simulink model "bare_system"  (Simulink 9.3)
settings: Solver=VariableStepAuto  StartTime=0.0  StopTime=stopTime  RelTol=1e-3
model workspace (MAT data in the model file):
  avg_usersArg = Simulink.Parameter
  avg_usersArg.Value = 4
  avg_usersArg.DataType = 'auto'
  avg_usersArg.Dimensions = [1 1]
  lambda1Arg = Simulink.Parameter
  lambda1Arg.Value = 1
  lambda1Arg.DataType = 'auto'
  lambda1Arg.Dimensions = [1 1]
  lambda2Arg = Simulink.Parameter
  lambda2Arg.Value = 1
  lambda2Arg.DataType = 'auto'
  lambda2Arg.Dimensions = [1 1]
  lower_limitArg = Simulink.Parameter
  lower_limitArg.Value = 1
  lower_limitArg.DataType = 'auto'
  lower_limitArg.Dimensions = [1 1]
  random_seedArg = Simulink.Parameter
  random_seedArg.Value = 1
  random_seedArg.DataType = 'auto'
  random_seedArg.Dimensions = [1 1]
  risk_delayArg = Simulink.Parameter
  risk_delayArg.Value = 1
  risk_delayArg.DataType = 'auto'
  risk_delayArg.Dimensions = [1 1]
  risk_delay_lengthArg = Simulink.Parameter
  risk_delay_lengthArg.Value = 1
  risk_delay_lengthArg.DataType = 'auto'
  risk_delay_lengthArg.Dimensions = [1 1]
  upper_limitArg = Simulink.Parameter
  upper_limitArg.Value = 1
  upper_limitArg.DataType = 'auto'
  upper_limitArg.Dimensions = [1 1]
values from neighbouring files (symbols this model uses):
  delta = 1e-10    [initParamsDefault.m]
  interval = 1    [train_ddpg.m]    (also in train_dqn.m)
  is_done_limit = 1200    [initParamsDefault.m]
  l1_cf = 2.4    [initParamsDefault.m]
  l1_ig = 1.5    [initParamsDefault.m]
  n = numel(vectors)    [initParamsDefault.m]
  omega = 0.1    [initParamsDefault.m]
  Pexec = 5    [initParamsDefault.m]
  Pidle = 0.1    [initParamsDefault.m]
  Ptx = 1    [initParamsDefault.m]
  Rate = [ ... (first row only)    [WIFI_speeds.m]
  sample_time = 0.1    [train_ddpg.m]    (also in train_dqn.m)
  stopTime = 40    [train_ddpg.m]    (also in train_dqn.m)
  tau_threshold = 5    [initParamsDefault.m]
  w_completion = 0.01    [initParamsDefault.m]
  w_drop = 1    [initParamsDefault.m]
  w_e = 0.5    [initParamsDefault.m]
  w_r = 1    [initParamsDefault.m]
  w_t = 0.1    [initParamsDefault.m]
undefined symbols (not defined in the file or in its folder): G11, G21, m
libraries: dspswit3 x2
settings Model: LogicAnalyzerSignalOrdering=7a861333-221d-4e7f-8add-257e68f24205,74d205a4-a193-4dc0-b1c9-8e90a76d10c0,8edb55ca-932c-4eaf-a437-d360681ad8d8,c1f7438e-c5c6-4b01-8a4c-5b6d5eaf2ff2,6056f5ae-7c1d-44d9-9ec1-3010ef70e335,fa087ba3-73e8-4d3e-98e3-f1da7fe23607,3810c5f4-a7a0-4a2b-8069-4553fd64eda7,c3949b75-f91e-4014-bb06-96fcff1975f8,1bed1f57-9200-4c38-84fd-82fc340e00e7,cf559684-595c-4874-ad9d-2b1e91fff60d,764e1eaf-4418-46bd-b041-cdf5e233247d,e1bf0d3d-4cd5-4e01-9ee8-80c20f0b8061,89db6489-1abe-4ea4-a088-9e6adbee9b0a,fb427c8a-da6d-4362-a6c5-a888e7a17672,bacb86b7-e896-464f-964b-2c73dcf349c9  Creator=Saurav  LastModifiedBy=Saurav  ParameterArgumentNames=lambda1Arg,lambda2Arg,random_seedArg,avg_usersArg,risk_delayArg,risk_delay_lengthArg,lower_limitArg,upper_limitArg
settings DataIOCC: SaveFormat=Dataset  SignalLoggingSaveFormat=Dataset  ReturnWorkspaceOutputs=on
settings OptimizationCC: LifeSpan=auto
settings DebuggingCC: UnderspecifiedInitializationDetection=Simplified  MergeDetectMultiDrivingBlocksExec=error  FcnCallInpInsideContextMsg=error  SFUnexpectedBacktrackingDiag=error  SFNoUnconditionalDefaultTransitionDiag=error  SFExecutionAtInitializationDiag=warning  ArithmeticOperatorsInVariantConditions=error
settings HardwareCC: ProdBitPerPointer=64  ProdBitPerSizeT=64  ProdBitPerPtrDiffT=64  ProdLargestAtomicFloat=Float  ProdIntDivRoundTo=Zero  ProdEndianess=LittleEndian  ProdWordSize=64  ProdHWDeviceType=Intel->x86-64 (Windows64)
settings ModelReferenceCC: PropagateSignalLabelsOutOfModel=on
settings SFSimCC: SimUseLocalCustomCode=on
settings RTWCC: RTWUseLocalCustomCode=on
settings CodeAppCC: StateflowObjectComments=off
settings GRTTargetCC: TargetLangStandard=C99 (ISO)  CombineOutputUpdateFcns=on  GRTInterface=off
settings ConfigComp: CovMetricSettings=dwe  CovHtmlReporting=off  CovSaveCumulativeToWorkspaceVar=off  CovSaveSingleToWorkspaceVar=off  CovExternalEMLEnable=on

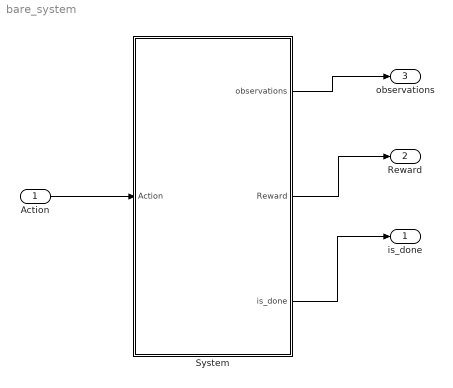
== system bare_system ==
  Action : Inport  SampleTime=interval
  System : Subsystem
  is_done : Outport  VectorParamsAs1DForOutWhenUnconnected=on
  Reward : Outport  Port=2  VectorParamsAs1DForOutWhenUnconnected=on
  observations : Outport  Port=3  SampleTime=interval  VectorParamsAs1DForOutWhenUnconnected=on
  wires:
  Action/1 -> System/1(Action)
  System/1(observations) -> observations/1
  System/2(Reward) -> Reward/1
  System/3(is_done) -> is_done/1

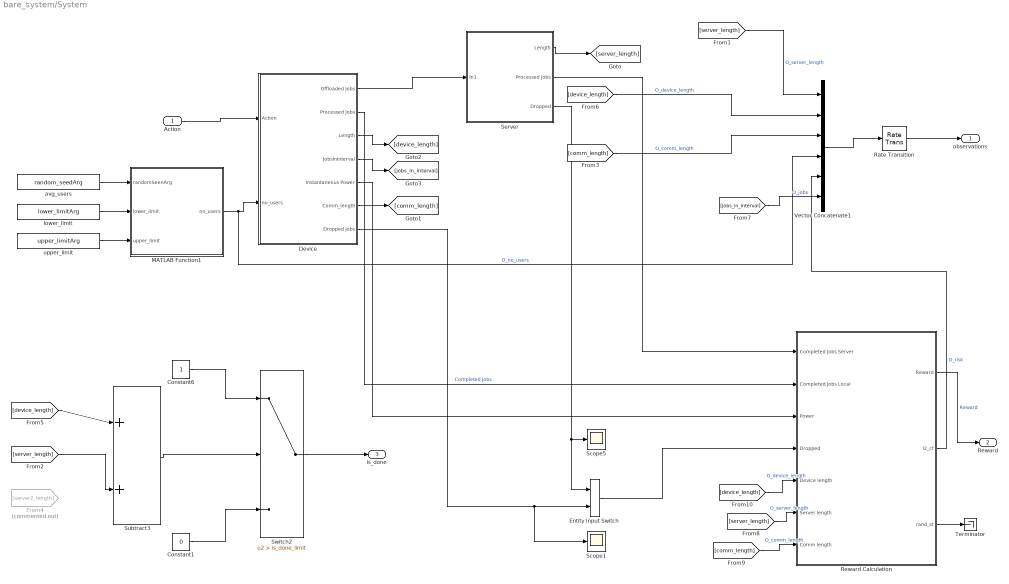
== system bare_system/System ==
  Action : Inport
  Constant1 : Constant  Value=0
  Constant6 : Constant
  Device : Subsystem
  Entity Input Switch : EntityInputSwitch  InputPortMessageModes=m,m  OutputPortMessageModes=m
  From4 : From  Commented=on  GotoTag=server2_length
  MATLAB Function1 : MATLAB Function  TreatAsAtomicUnit=on  SystemSampleTime=interval
  Rate Transition : RateTransition
  "Reward Calculation " : Subsystem
  Scope1 : Scope
  Scope5 : Scope
  Server : Subsystem  AncestorBlock=library/Server
  Subtract3 : Sum
  Switch2 : Switch  Criteria=u2 > Threshold  Threshold=is_done_limit
  Terminator : Terminator
  Vector Concatenate1 : Concatenate  NumInputs=6
  avg_users : Constant  Value=random_seedArg
  lower_limit : Constant  Value=lower_limitArg
  upper_limit : Constant  Value=upper_limitArg
  observations : Outport  SampleTime=interval  VectorParamsAs1DForOutWhenUnconnected=on
  Reward : Outport  Port=2  VectorParamsAs1DForOutWhenUnconnected=on
  is_done : Outport  Port=3  VectorParamsAs1DForOutWhenUnconnected=on
  wires:
  Device/5(Instantaneous Power) -> "Reward Calculation "/3(Power)
  Server/2(Processed Jobs) -> "Reward Calculation "/1(Completed Jobs Server)
  Device/6(Comm_length) -> [comm_length]
  Action/1 -> Device/1(Action)
  Constant1/1 -> Switch2/3
  Device/1(Offloaded Jobs) -> Server/1(In1)
  Server/1("Length ") -> [server_length]
  "Reward Calculation "/1(Reward) -> Reward/1  "Reward"
  Device/3("Length ") -> [device_length]
  Device/2(Processed Jobs) -> "Reward Calculation "/2(Completed Jobs Local)  "Completed Jobs"
  Device/4(JobsInInterval) -> [jobs_in_interval]
  [device_length] -> Subtract3/1
  Subtract3/1 -> Switch2/2
  Switch2/1 -> is_done/1
  [server_length] -> Subtract3/2
  Constant6/1 -> Switch2/1
  Device/7(Dropped Jobs) -> Scope1/1, Entity Input Switch/2
  Server/3(Dropped) -> Scope5/1, Entity Input Switch/1
  Entity Input Switch/1 -> "Reward Calculation "/4("Dropped ")
  Vector Concatenate1/1 -> Rate Transition/1
  Rate Transition/1 -> observations/1
  [device_length] -> "Reward Calculation "/5(Device length)  "O_device_length"
  [comm_length] -> "Reward Calculation "/7(Comm length)  "O_comm_length"
  [server_length] -> "Reward Calculation "/6(Server length)  "O_server_length"
  avg_users/1 -> MATLAB Function1/1(randomSeenArg)
  lower_limit/1 -> MATLAB Function1/2(lower_limit)
  upper_limit/1 -> MATLAB Function1/3(upper_limit)
  MATLAB Function1/1(no_users) -> Vector Concatenate1/4, Device/2("no_users ")  "O_no_users"
  [server_length] -> Vector Concatenate1/1  "O_server_length"
  [device_length] -> Vector Concatenate1/2  "O_device_length"
  [comm_length] -> Vector Concatenate1/3  "O_comm_length"
  "Reward Calculation "/2(l2_cf) -> Vector Concatenate1/5  "O_risk"
  "Reward Calculation "/3(rand_st) -> Terminator/1
  [jobs_in_interval] -> Vector Concatenate1/6  "O_jobs"

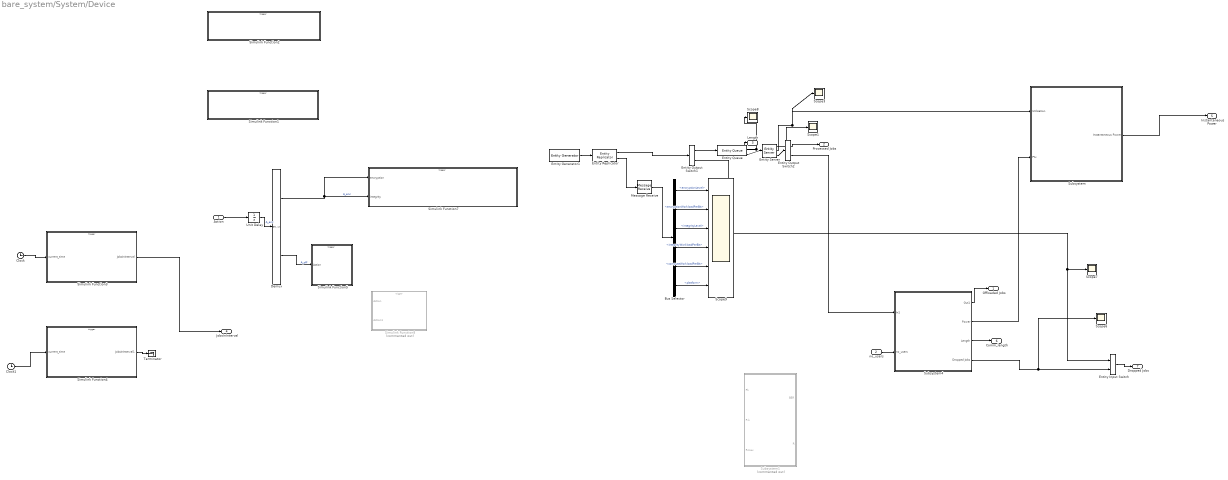
== system bare_system/System/Device ==
  Action : Inport
  "no_users " : Inport  Port=2
  Bus Selector : BusSelector  OutputSignals=encryptionLevel,encryptionWorkloadPerBit,integrityLevel,integrityWorkloadPerBit,computeWorkloadPerBit,platform
  Clock : Clock
  Clock1 : Clock
  Demux : Demux  Outputs=2
  Entity Input Switch : EntityInputSwitch  InputPortMessageModes=m,m  OutputPortMessageModes=m
  Entity Output Switch1 : EntityOutputSwitch  InputPortMessageModes=m  OutputPortMessageModes=m,m  SwitchAttributeName=platform
  Entity Output Switch2 : EntityOutputSwitch  InputPortMessageModes=m  OutputPortMessageModes=m,m  SwitchingCriterion=From attribute  SwitchAttributeName=platform
  Entity Generator1 : EntityGenerator  OutputPortMessageModes=m  TimeSource=MATLAB action  IntergenerationTimeAction=dt = predefinedArrivalTime();  GenerateEntityAtSimulationStart=off  GenerateAction=|  AttributeName=Size|GenerationTime  AttributeInitialValue=100|0  EntityType=Bus object  EntityTypeName=Job
      | entity.generationTime=stampEntity();
      | entity.size=j1_data_size; %200 kb
      | entity.id=idgenerator();
      | 
      | entity.computeWorkloadPerBit=j1_computeLoadPerBit;
      | [entity.encryptionLevel, entity.encryptionWorkloadPerBit,entity.integrityLevel, entity.integrityWorkloadPerBit] =selectSecurity();
      | entity.dropped=0;
      | % action=job1decision();
      | % r=rand();
      | % if (r<=action)
      | %     entity.platform=1;
      | % else
      | %     entity.platform=2;
      | % end
      | entity.platform=job1decision();
  Entity Queue : EntityQueue  InputPortMessageModes=m  OutputPortMessageModes=n,m  Capacity=20  NumberEntitiesInBlock=on
      settings: OutputPortMap=o1,o5
  Entity Replicator : EntityReplicator  InputPortMessageModes=m  OutputPortMessageModes=m,m
  Entity Server : EntityServer  InputPortMessageModes=m  OutputPortMessageModes=n,n,m  Capacity=device_cpu_cores  ServiceTimeSource=MATLAB action  ServiceTimeAction=|  AverageWait=on  Utilization=on
      | % Exponential service time with rate 1
      | % mean = 0.1;
      | if(entity.platform==1)
      |    wl=entity.computeWorkloadPerBit*entity.size; 
      |    
      | else
      |     wl=Im*(entity.encryptionWorkloadPerBit*entity.size+entity.integrityWorkloadPerBit*entity.size); 
      |     
      | end
      | dt=wl/Im;
      | 
      | % dt   = -average_computation_time_local * log(1 - rand());
      settings: OutputPortMap=o4,o5,o9
  Message Receive : MessageReceive  InputPortMessageModes=m
      settings: OutputPortMap=o1
  Scope{1,3,6..8} (5 alike) : Scope
  Scope9 : Scope  NumInputPorts=6
  Simulink Function1 : Subsystem  TreatAsAtomicUnit=on
  Simulink Function2 : Subsystem  TreatAsAtomicUnit=on
  Simulink Function3 : Subsystem  TreatAsAtomicUnit=on
  Simulink Function4 : Subsystem  TreatAsAtomicUnit=on
  Simulink Function5 : Subsystem  TreatAsAtomicUnit=on
  Simulink Function7 : Subsystem  TreatAsAtomicUnit=on
  Simulink Function8 : Subsystem  Commented=on  TreatAsAtomicUnit=on
  Subsystem : Subsystem
  Subsystem1 : Subsystem  Commented=on
  Subsystem4 : Subsystem
  Terminator : Terminator
  Unit Delay : UnitDelay  InitialCondition=[1 1]  SampleTime=-1  HasFrameUpgradeWarning=on
  Offloaded Jobs : Outport  VectorParamsAs1DForOutWhenUnconnected=on
  Processed Jobs : Outport  Port=2  VectorParamsAs1DForOutWhenUnconnected=on
  "Length " : Outport  Port=3  VectorParamsAs1DForOutWhenUnconnected=on
  JobsInInterval : Outport  Port=4  VectorParamsAs1DForOutWhenUnconnected=on
  Instantaneous Power : Outport  Port=5  VectorParamsAs1DForOutWhenUnconnected=on
  Comm_length : Outport  Port=6  VectorParamsAs1DForOutWhenUnconnected=on
  Dropped Jobs : Outport  Port=7  VectorParamsAs1DForOutWhenUnconnected=on
  wires:
  Clock/1 -> Simulink Function3/1(current_time)
  Subsystem/1(Instantaneous Power) -> Instantaneous Power/1
  Entity Server/2 -> Scope3/1, Subsystem/1(Utilisation)
  Entity Queue/2 -> Entity Server/1
  Simulink Function3/1(JobsInInterval) -> JobsInInterval/1
  Clock1/1 -> Simulink Function4/1(current_time)
  Entity Server/3 -> Entity Output Switch2/1
  Entity Output Switch2/1 -> Processed Jobs/1
  Subsystem4/1(Out1) -> Offloaded Jobs/1
  Subsystem4/2(Power) -> Subsystem/2(Ptx)
  Entity Output Switch2/2 -> Subsystem4/1(In1)
  "no_users "/1 -> Subsystem4/2("no_users ")
  Subsystem4/3("Length ") -> Comm_length/1
  Action/1 -> Unit Delay/1
  Simulink Function4/1(JobsInInterval1) -> Terminator/1
  Entity Output Switch1/1 -> Entity Queue/1
  Subsystem4/4(Dropped Jobs) -> Scope6/1, Entity Input Switch/2
  Entity Input Switch/1 -> Dropped Jobs/1
  Entity Server/1 -> Scope1/1
  Entity Queue/1 -> Scope8/1, "Length "/1
  Entity Output Switch1/2 -> Scope7/1, Entity Input Switch/1
  Entity Generator1/1 -> Entity Replicator/1
  Entity Replicator/1 -> Entity Output Switch1/1
  Entity Replicator/2 -> Message Receive/1
  Message Receive/1 -> Bus Selector/1
  Bus Selector/3 -> Scope9/3  "<integrityLevel>"
  Bus Selector/2 -> Scope9/2  "<encryptionWorkloadPerBit>"
  Bus Selector/4 -> Scope9/4  "<integrityWorkloadPerBit>"
  Bus Selector/1 -> Scope9/1  "<encryptionLevel>"
  Bus Selector/5 -> Scope9/5  "<computeWorkloadPerBit>"
  Bus Selector/6 -> Scope9/6  "<platform>"
  Unit Delay/1 -> Demux/1  "A_enc"
  Demux/1 -> Simulink Function7/2(integrity), Simulink Function7/1(encryption)  "A_enc"
  Demux/2 -> Simulink Function5/1(Action)  "A_off"

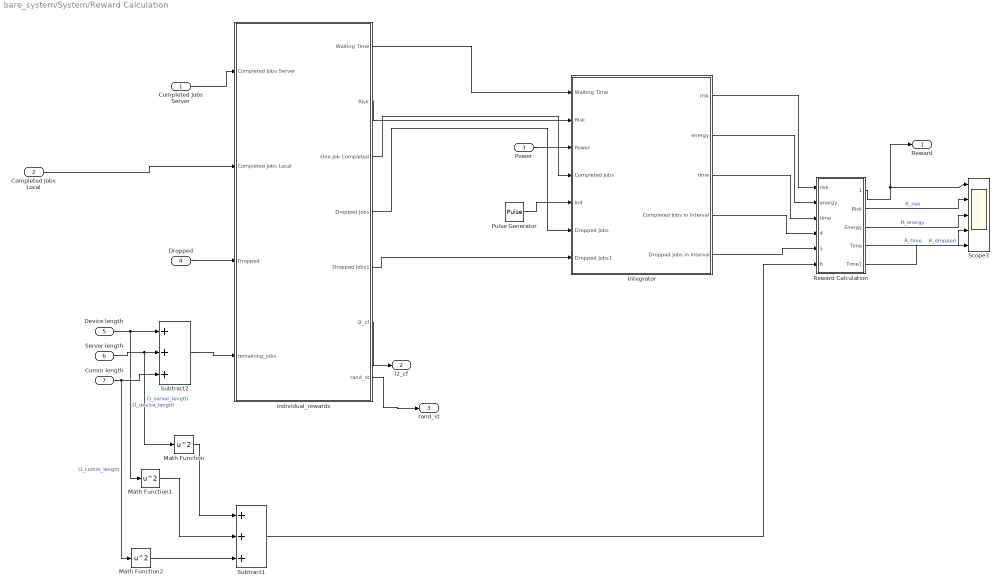
== system bare_system/System/Reward Calculation  ==
  Completed Jobs Server : Inport
  Completed Jobs Local : Inport  Port=2
  Power : Inport  Port=3
  "Dropped " : Inport  Port=4
  Device length : Inport  Port=5
  Server length : Inport  Port=6
  Comm length : Inport  Port=7
  Integrator : Subsystem
  Math Function : Math  Operator=square  SaturateOnIntegerOverflow=on
  Math Function1 : Math  Operator=square  SaturateOnIntegerOverflow=on
  Math Function2 : Math  Operator=square  SaturateOnIntegerOverflow=on
  Pulse Generator : DiscretePulseGenerator  PulseType=Time based  Period=interval
  Reward Calculation : Subsystem  TreatAsAtomicUnit=on  SystemSampleTime=interval
  Scope3 : Scope  NumInputPorts=5
  Subtract1 : Sum  Inputs=+++
  Subtract2 : Sum  Inputs=+++
  individual_rewards : Subsystem
  Reward : Outport  VectorParamsAs1DForOutWhenUnconnected=on
  l2_cf : Outport  Port=2  VectorParamsAs1DForOutWhenUnconnected=on
  rand_st : Outport  Port=3  VectorParamsAs1DForOutWhenUnconnected=on
  wires:
  Integrator/4(Completed Jobs in Interval) -> Reward Calculation/4(Completed Jobs)
  Integrator/5(Dropped Jobs in Interval) -> Reward Calculation/5(Dropped Jobs)
  Integrator/3(time) -> Reward Calculation/3(time)
  Integrator/2(energy) -> Reward Calculation/2(energy)
  Reward Calculation/2(Risk) -> Scope3/2  "R_risk"
  Reward Calculation/3(Energy) -> Scope3/3  "R_energy"
  Reward Calculation/4(Time) -> Scope3/4  "R_time"
  Integrator/1(risk) -> Reward Calculation/1(risk)
  Pulse Generator/1 -> Integrator/5(In4)
  Power/1 -> Integrator/3(Power)
  individual_rewards/1(Waiting Time) -> Integrator/1(Waiting Time)
  Reward Calculation/1(Reward) -> Reward/1, Scope3/1
  Completed Jobs Server/1 -> individual_rewards/1(Completed Jobs Server)
  individual_rewards/2(Risk) -> Integrator/2(Risk)
  individual_rewards/3(One Job Completed) -> Integrator/4(Completed Jobs)
  "Dropped "/1 -> individual_rewards/3("Dropped ")
  individual_rewards/4(Dropped Jobs) -> Integrator/6(Dropped Jobs)
  individual_rewards/5(Dropped Jobs1) -> Integrator/7(Dropped Jobs1)
  Reward Calculation/5(Time1) -> Scope3/5  "R_dropped"
  Completed Jobs Local/1 -> individual_rewards/2(Completed Jobs Local)
  Subtract1/1 -> Reward Calculation/6("remaining_jobs ")
  Subtract2/1 -> individual_rewards/4("remaining_jobs ")
  Server length/1 -> Math Function/1, Subtract2/2  "O_server_length"
  Math Function1/1 -> Subtract1/2
  Device length/1 -> Math Function1/1, Subtract2/1  "O_device_length"
  Math Function2/1 -> Subtract1/3
  Comm length/1 -> Math Function2/1, Subtract2/3  "O_comm_length"
  Math Function/1 -> Subtract1/1
  individual_rewards/6(l2_cf) -> l2_cf/1
  individual_rewards/7(rand_st) -> rand_st/1

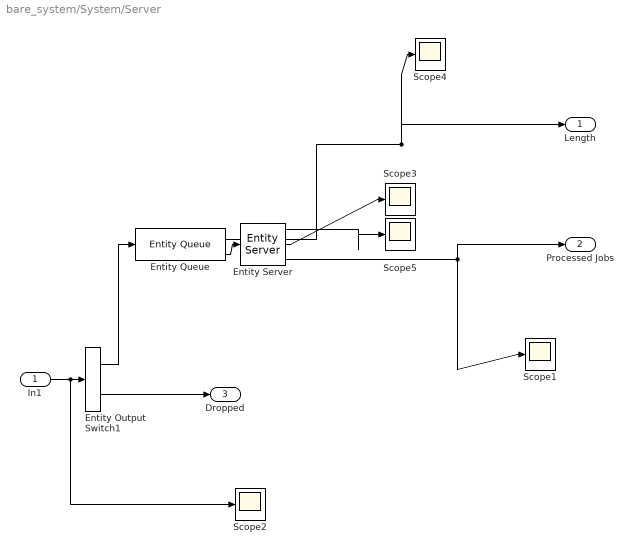
== system bare_system/System/Server ==
  In1 : Inport
  Entity Output Switch1 : EntityOutputSwitch  InputPortMessageModes=m  OutputPortMessageModes=m,m  SwitchAttributeName=platform
  Entity Queue : EntityQueue  InputPortMessageModes=m  OutputPortMessageModes=n,m  Capacity=10  NumberEntitiesInBlock=on
      settings: OutputPortMap=o1,o5
  Entity Server : EntityServer  InputPortMessageModes=m  OutputPortMessageModes=n,n,m  Capacity=server_cpu_cores  ServiceTimeSource=MATLAB action  ServiceTimeAction=|  NumberEntitiesDeparted=on  Utilization=on
      | % Exponential service time with rate 1
      | % mean = 0.1;
      | % dt   = -average_computation_time_server * log(1 - rand());
      | 
      | % if(entity.platform==2)
      |     % decryption
      |    wl=Is*(entity.encryptionWorkloadPerBit*entity.size+entity.integrityWorkloadPerBit*entity.size) +entity.computeWorkloadPerBit*entity.size;
      | % else
      | %     wl=1;
      | %     disp('I shouldn not be here');
      | % end
      | dt=wl/Is;
      settings: OutputPortMap=o0,o5,o9
  Scope{1..5} (5 alike) : Scope
  "Length " : Outport  VectorParamsAs1DForOutWhenUnconnected=on
  Processed Jobs : Outport  Port=2  VectorParamsAs1DForOutWhenUnconnected=on
  Dropped : Outport  Port=3  VectorParamsAs1DForOutWhenUnconnected=on
  wires:
  Entity Server/3 -> Scope1/1, Processed Jobs/1
  Entity Queue/1 -> Scope4/1, "Length "/1
  Entity Queue/2 -> Entity Server/1
  In1/1 -> Scope2/1, Entity Output Switch1/1
  Entity Output Switch1/1 -> Entity Queue/1
  Entity Output Switch1/2 -> Dropped/1
  Entity Server/2 -> Scope3/1
  Entity Server/1 -> Scope5/1

== system bare_system/System/Device/Simulink Function1 ==
  idgenerator : TriggerPort  TriggerType=function-call  IsSimulinkFunction=on  FunctionName=idgenerator  VariantControl=Variant
  MATLAB Function : MATLAB Function  TreatAsAtomicUnit=on
  id : ArgOut  DisableCoverage=on  ArgumentName=id
  wires:
  MATLAB Function/1(idx) -> id/1

== system bare_system/System/Device/Simulink Function2 ==
  stampEntity : TriggerPort  TriggerType=function-call  IsSimulinkFunction=on  FunctionName=stampEntity  VariantControl=Variant
  Digital Clock : DigitalClock  SampleTime=-1
  t : ArgOut  DisableCoverage=on  ArgumentName=t
  wires:
  Digital Clock/1 -> t/1

== system bare_system/System/Device/Simulink Function3 ==
  current_time : Inport
  predefinedArrivalTime : TriggerPort  TriggerType=function-call  IsSimulinkFunction=on  FunctionName=predefinedArrivalTime  VariantControl=Variant
  Arrival Rate2 : Constant  Value=interval  SampleTime=-1
  MATLAB Function : MATLAB Function  TreatAsAtomicUnit=on
  Scope1 : Scope
  Scope2 : Scope
  Scope5 : Scope
  lambda1 : Constant  Value=lambda1Arg  SampleTime=-1
  random_seed : Constant  Value=random_seedArg  SampleTime=-1
  stopTime : Constant  Value=stopTime  SampleTime=-1
  t1 : ArgOut  DisableCoverage=on  ArgumentName=t
  JobsInInterval : Outport  VectorParamsAs1DForOutWhenUnconnected=on
  wires:
  random_seed/1 -> Scope1/1, MATLAB Function/5(seed)
  lambda1/1 -> Scope2/1, MATLAB Function/1(l1)
  Arrival Rate2/1 -> MATLAB Function/3(interval)
  stopTime/1 -> MATLAB Function/2(total_time)
  current_time/1 -> MATLAB Function/4(curr_time)
  MATLAB Function/1(dt) -> Scope5/1, t1/1
  MATLAB Function/2(j1_in) -> JobsInInterval/1

== system bare_system/System/Device/Simulink Function4 ==
  current_time : Inport
  predefinedArrivalTime2 : TriggerPort  TriggerType=function-call  IsSimulinkFunction=on  FunctionName=predefinedArrivalTime2  VariantControl=Variant
  Arrival Rate2 : Constant  Value=interval  SampleTime=-1
  MATLAB Function : MATLAB Function  TreatAsAtomicUnit=on
  Scope1 : Scope
  lambda2 : Constant  Value=lambda2Arg  SampleTime=-1
  stopTime : Constant  Value=stopTime  SampleTime=-1
  t : ArgOut  DisableCoverage=on  ArgumentName=t
  JobsInInterval1 : Outport  VectorParamsAs1DForOutWhenUnconnected=on
  wires:
  MATLAB Function/2(j2_in) -> JobsInInterval1/1
  MATLAB Function/1(dt) -> t/1, Scope1/1
  current_time/1 -> MATLAB Function/4(curr_time)
  lambda2/1 -> MATLAB Function/1(l2)
  stopTime/1 -> MATLAB Function/2(total_time)
  Arrival Rate2/1 -> MATLAB Function/3(interval)

== system bare_system/System/Device/Simulink Function5 ==
  Action : Inport
  job1decision : TriggerPort  TriggerType=function-call  IsSimulinkFunction=on  FunctionName=job1decision  FunctionVisibility=scoped  VariantControl=(inherit)
  MATLAB Function2 : MATLAB Function  TreatAsAtomicUnit=on
  offload : ArgOut  DisableCoverage=on  ArgumentName=platform
  wires:
  Action/1 -> MATLAB Function2/1(action1)
  MATLAB Function2/1(platform) -> offload/1

== system bare_system/System/Device/Simulink Function7 ==
  encryption : Inport
  integrity : Inport  Port=2
  selectSecurity : TriggerPort  TriggerType=function-call  IsSimulinkFunction=on  FunctionName=selectSecurity  FunctionVisibility=scoped  VariantControl=(inherit)
  MATLAB Function2 : MATLAB Function  TreatAsAtomicUnit=on
  encryptionLevel : ArgOut  DisableCoverage=on  ArgumentName=encryptionLevel
  encryptionWorkloadPerBit : ArgOut  DisableCoverage=on  Port=2  ArgumentName=encryptionWorkloadPerBit
  integrityLevel : ArgOut  DisableCoverage=on  Port=3  ArgumentName=integrityLevel
  integrityWorkloadPerBit : ArgOut  DisableCoverage=on  Port=4  ArgumentName=integrityWorkloadPerBit
  wires:
  encryption/1 -> MATLAB Function2/1("encryptionLevel ")
  MATLAB Function2/1(encryptionLevel) -> encryptionLevel/1
  MATLAB Function2/2(encryptionWorkloadPerBit) -> encryptionWorkloadPerBit/1
  MATLAB Function2/3(integrityLevel) -> integrityLevel/1
  MATLAB Function2/4(integrityWorkloadPerBit) -> integrityWorkloadPerBit/1
  integrity/1 -> MATLAB Function2/2("integrityLevel ")

== system bare_system/System/Device/Simulink Function8 ==
  Action : Inport
  Action1 : Inport  Port=2
  job2decision : TriggerPort  TriggerType=function-call  IsSimulinkFunction=on  FunctionName=job2decision  FunctionVisibility=scoped  VariantControl=(inherit)
  MATLAB Function2 : MATLAB Function  TreatAsAtomicUnit=on
  offload : ArgOut  DisableCoverage=on  ArgumentName=platform
  wires:
  Action1/1 -> MATLAB Function2/2(action2)
  Action/1 -> MATLAB Function2/1(action1)
  MATLAB Function2/1(platform) -> offload/1

== system bare_system/System/Device/Subsystem ==
  Utilisation : Inport
  Ptx : Inport  Port=2
  Constant1 : Constant
  Constant2 : Constant  Value=Pidle
  Constant4 : Constant  Value=Pexec
  Divide : Product  Inputs=**
  Divide1 : Product  Inputs=**
  Subtract1 : Sum  Inputs=+-
  add : Sum  Inputs=+++
  Instantaneous Power : Outport  VectorParamsAs1DForOutWhenUnconnected=on
  wires:
  Constant4/1 -> Divide/1
  Constant1/1 -> Subtract1/1
  add/1 -> Instantaneous Power/1
  Subtract1/1 -> Divide1/2
  Divide/1 -> add/2
  Constant2/1 -> Divide1/1
  Divide1/1 -> add/1
  Utilisation/1 -> Subtract1/2, Divide/2
  Ptx/1 -> add/3

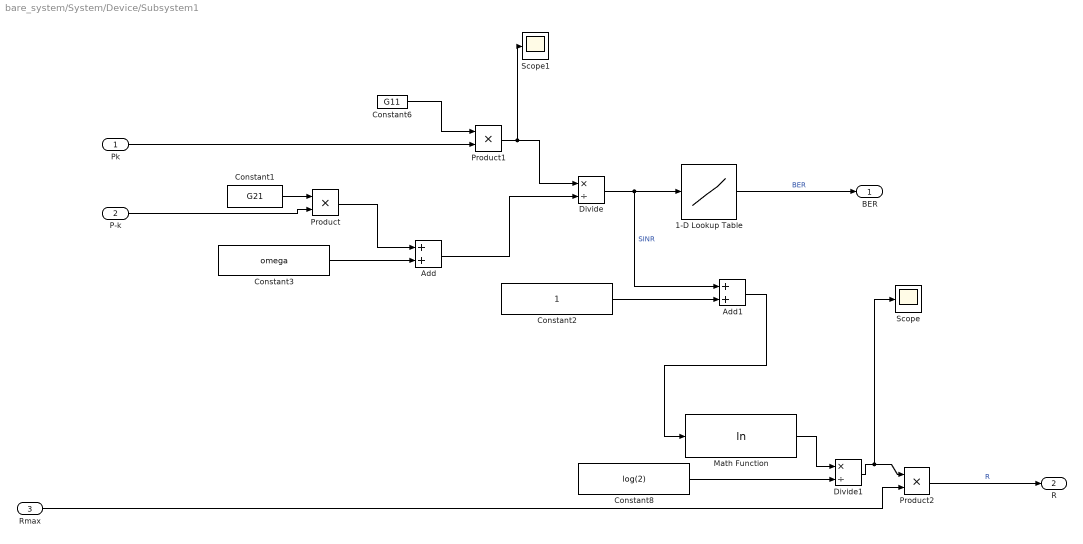
== system bare_system/System/Device/Subsystem1 ==
  Pk : Inport
  P-k : Inport  Port=2
  Rmax : Inport  Port=3
  1-D Lookup Table : Lookup_n-D  NumberOfTableDimensions=1  BreakpointsForDimension1=[-5:5]  Table=tanh([-5:5])  InternalRulePriority=Speed  RndMeth=Simplest  InputSameDT=on
  Add : Sum
  Add1 : Sum
  Constant1 : Constant  Value=G21
  Constant2 : Constant
  Constant3 : Constant  Value=omega
  Constant6 : Constant  Value=G11
  Constant8 : Constant  Value=log(2)
  Divide : Product  Inputs=*/
  Divide1 : Product  Inputs=*/
  Math Function : Math  Operator=log  SaturateOnIntegerOverflow=on
  Product : Product
  Product1 : Product
  Product2 : Product
  Scope : Scope
  Scope1 : Scope
  BER : Outport  VectorParamsAs1DForOutWhenUnconnected=on
  R : Outport  Port=2  VectorParamsAs1DForOutWhenUnconnected=on
  wires:
  Divide1/1 -> Scope/1, Product2/1
  1-D Lookup Table/1 -> BER/1  "BER"
  Constant8/1 -> Divide1/2
  Math Function/1 -> Divide1/1
  Add1/1 -> Math Function/1
  Constant2/1 -> Add1/2
  Product1/1 -> Divide/1, Scope1/1
  Product2/1 -> R/1  "R"
  Constant1/1 -> Product/1
  Constant3/1 -> Add/2
  Constant6/1 -> Product1/1
  Divide/1 -> Add1/1, 1-D Lookup Table/1  "SINR"
  Pk/1 -> Product1/2
  Add/1 -> Divide/2
  P-k/1 -> Product/2
  Rmax/1 -> Product2/2
  Product/1 -> Add/1

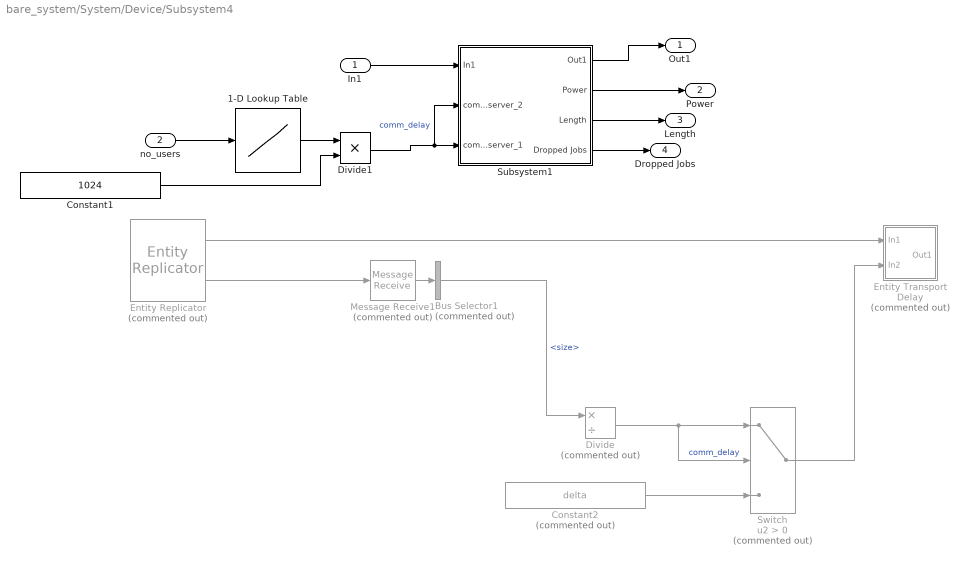
== system bare_system/System/Device/Subsystem4 ==
  In1 : Inport
  "no_users " : Inport  Port=2
  1-D Lookup Table : Lookup_n-D  NumberOfTableDimensions=1  BreakpointsForDimension1=[1:100]  Table=Rate  InternalRulePriority=Speed  RndMeth=Simplest  InputSameDT=on
  Bus Selector1 : BusSelector  Commented=on  OutputSignals=size
  Constant1 : Constant  Value=1024
  Constant2 : Constant  Commented=on  Value=delta
  Divide : Product  Commented=on  Inputs=*/
  Divide1 : Product  Inputs=**
  Entity Transport Delay : Subsystem  Description=Replaced Block  Commented=on  mask(Replaced Block){}
      mask help: This block has been replaced with an empty subsystem because it used functionality that is unavailable in Simulink R2019a.
      mask Display: fprintf('Replaced: %s\n','EntityTransportDelay')
  Entity Replicator : EntityReplicator  Commented=on  InputPortMessageModes=m  OutputPortMessageModes=m,m
  Message Receive1 : MessageReceive  Commented=on  InputPortMessageModes=m  ValueSourceWhenQueueIsEmpty=Use initial value
      settings: OutputPortMap=o1
  Subsystem1 : Subsystem
  Switch : Switch  Commented=on  Criteria=u2 > Threshold
  Out1 : Outport  VectorParamsAs1DForOutWhenUnconnected=on
  Power : Outport  Port=2  VectorParamsAs1DForOutWhenUnconnected=on
  "Length " : Outport  Port=3  VectorParamsAs1DForOutWhenUnconnected=on
  Dropped Jobs : Outport  Port=4  VectorParamsAs1DForOutWhenUnconnected=on
  wires:
  "no_users "/1 -> 1-D Lookup Table/1
  Constant2/1 -> Switch/3
  Switch/1 -> Entity Transport Delay/2(In2)
  Entity Replicator/2 -> Message Receive1/1
  Divide/1 -> Switch/1, Switch/2  "comm_delay"
  Bus Selector1/1 -> Divide/1  "<size>"
  Message Receive1/1 -> Bus Selector1/1
  Entity Replicator/1 -> Entity Transport Delay/1(In1)
  1-D Lookup Table/1 -> Divide1/1
  Constant1/1 -> Divide1/2
  In1/1 -> Subsystem1/1(In1)
  Divide1/1 -> Subsystem1/2(comm_delay_server_2), Subsystem1/3(comm_delay_server_1)  "comm_delay"
  Subsystem1/1(Out1) -> Out1/1
  Subsystem1/2(Power) -> Power/1
  Subsystem1/3("Length ") -> "Length "/1
  Subsystem1/4(Dropped Jobs) -> Dropped Jobs/1

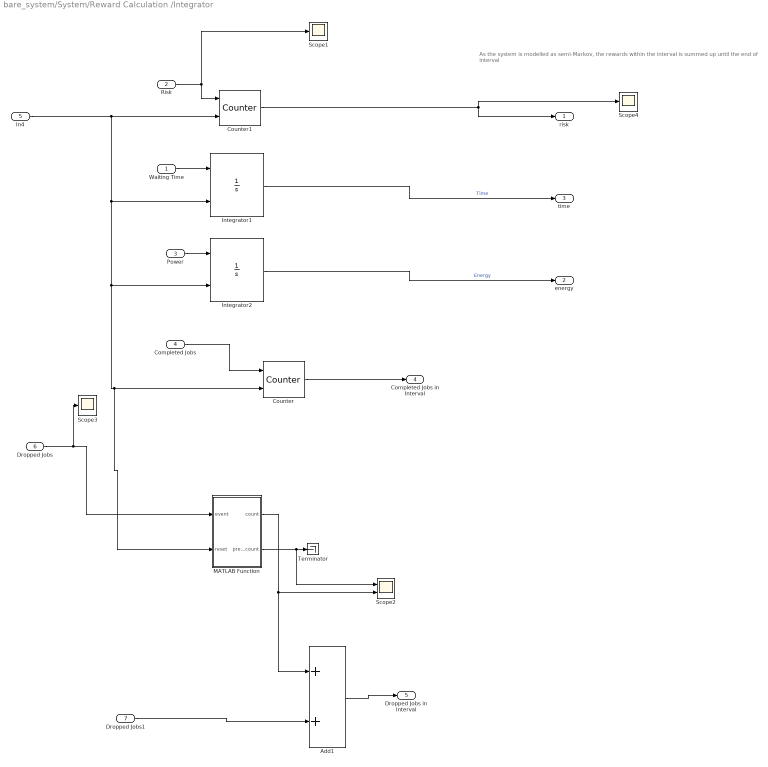
== system bare_system/System/Reward Calculation /Integrator ==
  note: As the system is modelled as semi-Markov, the rewards within the interval is summed up until the end of interval
  Waiting Time : Inport
  Risk : Inport  Port=2
  Power : Inport  Port=3
  Completed Jobs : Inport  Port=4
  In4 : Inport  Port=5
  Dropped Jobs : Inport  Port=6
  Dropped Jobs1 : Inport  Port=7
  Add1 : Sum
  Counter : dspswit3/Counter  Direction=Up  CountEvent=Falling edge  CounterSize=User defined  MaxCount=1000  InitialCount=0  Output=Count  HitValue=32  ResetInput=on  SamplesPerFrame=1  Ts=1  CntDtype=double  HitDtype=Logical
  Counter1 : dspswit3/Counter  Direction=Up  CountEvent=Falling edge  CounterSize=User defined  MaxCount=1000  InitialCount=0  Output=Count  HitValue=32  ResetInput=on  SamplesPerFrame=1  Ts=1  CntDtype=double  HitDtype=Logical
  Integrator1 : Integrator  ExternalReset=falling
  Integrator2 : Integrator  ExternalReset=falling
  MATLAB Function : MATLAB Function  TreatAsAtomicUnit=on  SystemSampleTime=sample_time
  Scope1 : Scope
  Scope2 : Scope  NumInputPorts=2
  Scope3 : Scope
  Scope4 : Scope
  Terminator : Terminator
  risk : Outport  VectorParamsAs1DForOutWhenUnconnected=on
  energy : Outport  Port=2  VectorParamsAs1DForOutWhenUnconnected=on
  time : Outport  Port=3  VectorParamsAs1DForOutWhenUnconnected=on
  Completed Jobs in Interval : Outport  Port=4  VectorParamsAs1DForOutWhenUnconnected=on
  Dropped Jobs in Interval : Outport  Port=5  VectorParamsAs1DForOutWhenUnconnected=on
  wires:
  Waiting Time/1 -> Integrator1/1
  Risk/1 -> Counter1/1, Scope1/1
  Power/1 -> Integrator2/1
  In4/1 -> Counter1/2, MATLAB Function/2(reset), Counter/2, Integrator2/2, Integrator1/2
  Integrator1/1 -> time/1  "Time"
  Integrator2/1 -> energy/1  "Energy"
  Completed Jobs/1 -> Counter/1
  Counter/1 -> Completed Jobs in Interval/1
  Counter1/1 -> Scope4/1, risk/1
  Dropped Jobs/1 -> Scope3/1, MATLAB Function/1(event)
  MATLAB Function/1(count) -> Add1/1, Scope2/2
  MATLAB Function/2(prev_count) -> Scope2/1, Terminator/1
  Dropped Jobs1/1 -> Add1/2
  Add1/1 -> Dropped Jobs in Interval/1

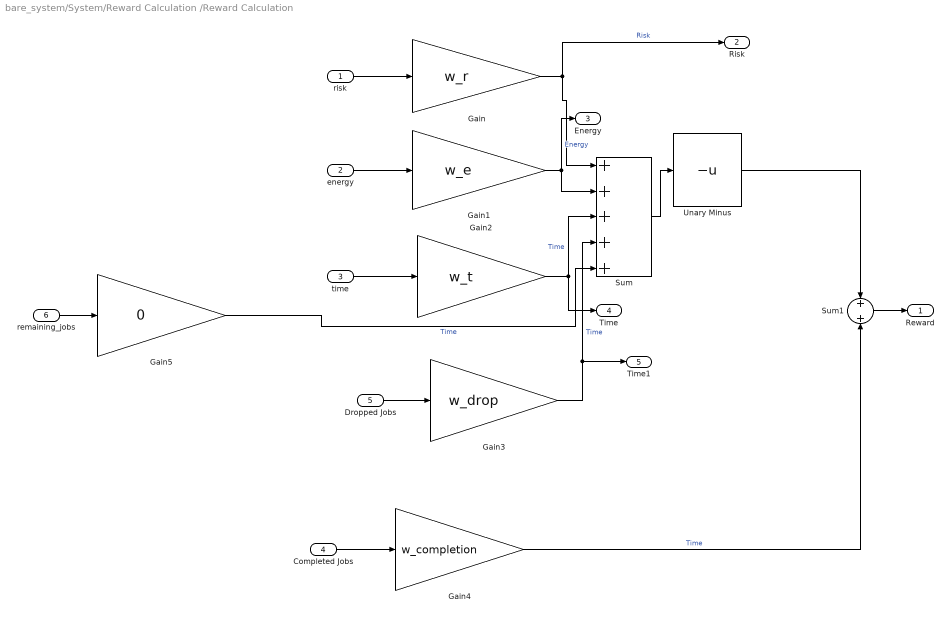
== system bare_system/System/Reward Calculation /Reward Calculation ==
  risk : Inport
  energy : Inport  Port=2
  time : Inport  Port=3
  Completed Jobs : Inport  Port=4
  Dropped Jobs : Inport  Port=5
  "remaining_jobs " : Inport  Port=6
  Gain : Gain  Gain=w_r
  Gain1 : Gain  Gain=w_e
  Gain2 : Gain  Gain=w_t
  Gain3 : Gain  Gain=w_drop
  Gain4 : Gain  Gain=w_completion
  Gain5 : Gain  Gain=0
  Sum : Sum  Inputs=+++++
  Sum1 : Sum
  Unary Minus : UnaryMinus
  Reward : Outport  VectorParamsAs1DForOutWhenUnconnected=on
  Risk : Outport  Port=2  VectorParamsAs1DForOutWhenUnconnected=on
  Energy : Outport  Port=3  VectorParamsAs1DForOutWhenUnconnected=on
  Time : Outport  Port=4  VectorParamsAs1DForOutWhenUnconnected=on
  Time1 : Outport  Port=5  VectorParamsAs1DForOutWhenUnconnected=on
  wires:
  Gain3/1 -> Time1/1, Sum/4  "Time"
  Dropped Jobs/1 -> Gain3/1
  time/1 -> Gain2/1
  energy/1 -> Gain1/1
  risk/1 -> Gain/1
  Gain1/1 -> Sum/2, Energy/1  "Energy"
  Gain/1 -> Sum/1, Risk/1  "Risk"
  Sum/1 -> Unary Minus/1
  Gain2/1 -> Sum/3, Time/1  "Time"
  Unary Minus/1 -> Sum1/1
  Gain4/1 -> Sum1/2  "Time"
  Sum1/1 -> Reward/1
  Completed Jobs/1 -> Gain4/1
  "remaining_jobs "/1 -> Gain5/1
  Gain5/1 -> Sum/5  "Time"

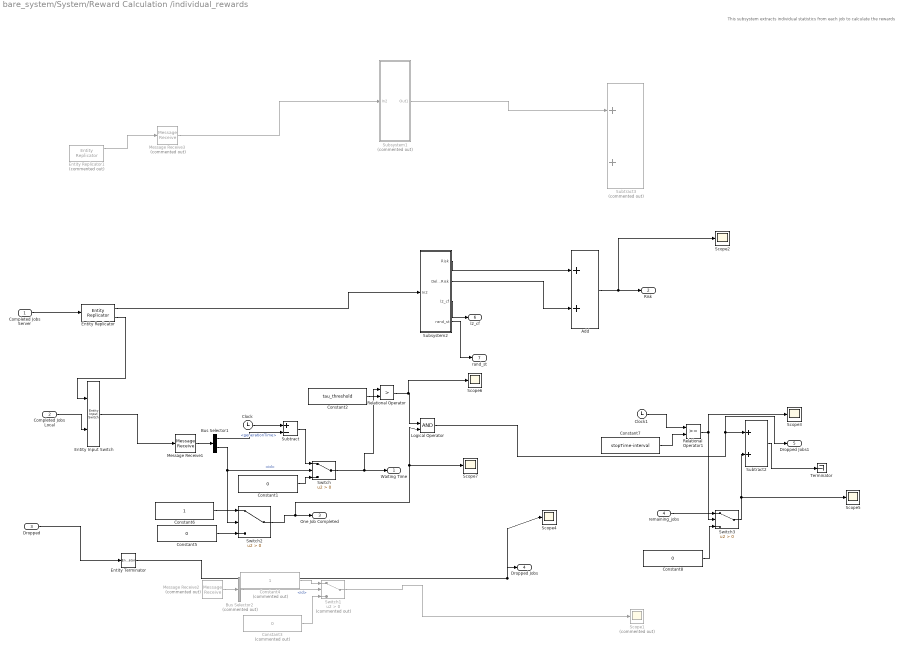
== system bare_system/System/Reward Calculation /individual_rewards ==
  note: This subsystem extracts individual statistics from each job to calculate the rewards
  Completed Jobs Server : Inport
  Completed Jobs Local : Inport  Port=2
  "Dropped " : Inport  Port=3
  "remaining_jobs " : Inport  Port=4
  Add : Sum
  Bus Selector1 : BusSelector  OutputSignals=generationTime,id
  Bus Selector2 : BusSelector  Commented=on  OutputSignals=id
  Clock : Clock
      settings: Decimation=1/sample_time
  Clock1 : Clock
      settings: Decimation=1/sample_time
  Constant1 : Constant  Value=0
  Constant2 : Constant  Value=tau_threshold
  Constant3 : Constant  Commented=on  Value=0
  Constant4 : Constant  Commented=on
  Constant5 : Constant  Value=0
  Constant6 : Constant
  Constant7 : Constant  Value=stopTime-interval
  Constant8 : Constant  Value=0
  Entity Input Switch : EntityInputSwitch  InputPortMessageModes=m,m  OutputPortMessageModes=m
  Entity Replicator : EntityReplicator  InputPortMessageModes=m  OutputPortMessageModes=m,m
  Entity Replicator1 : EntityReplicator  Commented=on  InputPortMessageModes=m  OutputPortMessageModes=m,m
  Entity Terminator : EntityTerminator  InputPortMessageModes=m  NumberEntitiesArrived=on
      settings: OutputPortMap=o0
  Logical Operator : Logic  IconShape=distinctive  AllPortsSameDT=off  OutDataTypeStr=boolean
  Message Receive1 : MessageReceive  InputPortMessageModes=m  ValueSourceWhenQueueIsEmpty=Use initial value  SampleTime=sample_time
      settings: OutputPortMap=o1
  Message Receive2 : MessageReceive  Commented=on  InputPortMessageModes=m  ValueSourceWhenQueueIsEmpty=Use initial value  SampleTime=sample_time
      settings: OutputPortMap=o1
  Message Receive3 : MessageReceive  Commented=on  InputPortMessageModes=m  ValueSourceWhenQueueIsEmpty=Use initial value
      settings: OutputPortMap=o1
  Relational Operator : RelationalOperator  Operator=>  OutDataTypeStr=boolean  RndMeth=Simplest
  Relational Operator1 : RelationalOperator  OutDataTypeStr=boolean  RndMeth=Simplest
  Scope1 : Scope  Commented=on
  Scope{2..7} (6 alike) : Scope
  Subsystem1 : Subsystem  Commented=on
  Subsystem2 : Subsystem
  Subtract : Sum  Inputs=+-
  Subtract2 : Sum
  Subtract3 : Sum  Commented=on
  Switch : Switch  Criteria=u2 > Threshold
  Switch1 : Switch  Commented=on  Criteria=u2 > Threshold
  Switch2 : Switch  Criteria=u2 > Threshold
  Switch3 : Switch  Criteria=u2 > Threshold
  Terminator : Terminator
  Waiting Time : Outport  VectorParamsAs1DForOutWhenUnconnected=on
  Risk : Outport  Port=2  VectorParamsAs1DForOutWhenUnconnected=on
  One Job Completed : Outport  Port=3  VectorParamsAs1DForOutWhenUnconnected=on
  Dropped Jobs : Outport  Port=4  VectorParamsAs1DForOutWhenUnconnected=on
  Dropped Jobs1 : Outport  Port=5  VectorParamsAs1DForOutWhenUnconnected=on
  l2_cf : Outport  Port=6  VectorParamsAs1DForOutWhenUnconnected=on
  rand_st : Outport  Port=7  VectorParamsAs1DForOutWhenUnconnected=on
  wires:
  Relational Operator/1 -> Scope6/1, Logical Operator/1
  Constant2/1 -> Relational Operator/2
  Subsystem1/1(Out1) -> Subtract3/1
  Message Receive3/1 -> Subsystem1/1(In2)
  Entity Replicator1/1 -> Message Receive3/1
  Entity Replicator/1 -> Subsystem2/1(In2)
  Switch2/1 -> Scope7/1, Logical Operator/2, One Job Completed/1
  Subtract/1 -> Switch/1
  Switch/1 -> Relational Operator/1, Waiting Time/1
  Clock/1 -> Subtract/1
  Message Receive1/1 -> Bus Selector1/1
  Completed Jobs Local/1 -> Entity Input Switch/2
  Completed Jobs Server/1 -> Entity Replicator/1
  Entity Replicator/2 -> Entity Input Switch/1
  Bus Selector1/2 -> Switch/2, Switch2/2  "<id>"
  Constant5/1 -> Switch2/3
  Constant6/1 -> Switch2/1
  Constant1/1 -> Switch/3
  Bus Selector1/1 -> Subtract/2  "<generationTime>"
  Subsystem2/2(Delayed Risk) -> Add/2
  Subsystem2/1(Risk) -> Add/1
  Add/1 -> Scope2/1, Risk/1
  Message Receive2/1 -> Bus Selector2/1
  Constant3/1 -> Switch1/3
  Constant4/1 -> Switch1/1
  Bus Selector2/1 -> Switch1/2  "<id>"
  Switch1/1 -> Scope1/1
  Entity Input Switch/1 -> Message Receive1/1
  "Dropped "/1 -> Entity Terminator/1
  Entity Terminator/1 -> Scope4/1, Dropped Jobs/1
  Switch3/1 -> Subtract2/2, Scope5/1
  Logical Operator/1 -> Dropped Jobs1/1, Subtract2/1
  Constant8/1 -> Switch3/3
  Relational Operator1/1 -> Scope3/1, Switch3/2
  "remaining_jobs "/1 -> Switch3/1
  Constant7/1 -> Relational Operator1/2
  Clock1/1 -> Relational Operator1/1
  Subtract2/1 -> Terminator/1
  Subsystem2/3(l2_cf) -> l2_cf/1
  Subsystem2/4(rand_st) -> rand_st/1

== system bare_system/System/Device/Subsystem4/Entity Transport Delay ==
  In1 : Inport
  In2 : Inport  Port=2
  Ground1 : Ground
  Terminator1 : Terminator
  Terminator2 : Terminator
  Out1 : Outport  VectorParamsAs1DForOutWhenUnconnected=on
  wires:
  Ground1/1 -> Out1/1
  In2/1 -> Terminator2/1
  In1/1 -> Terminator1/1

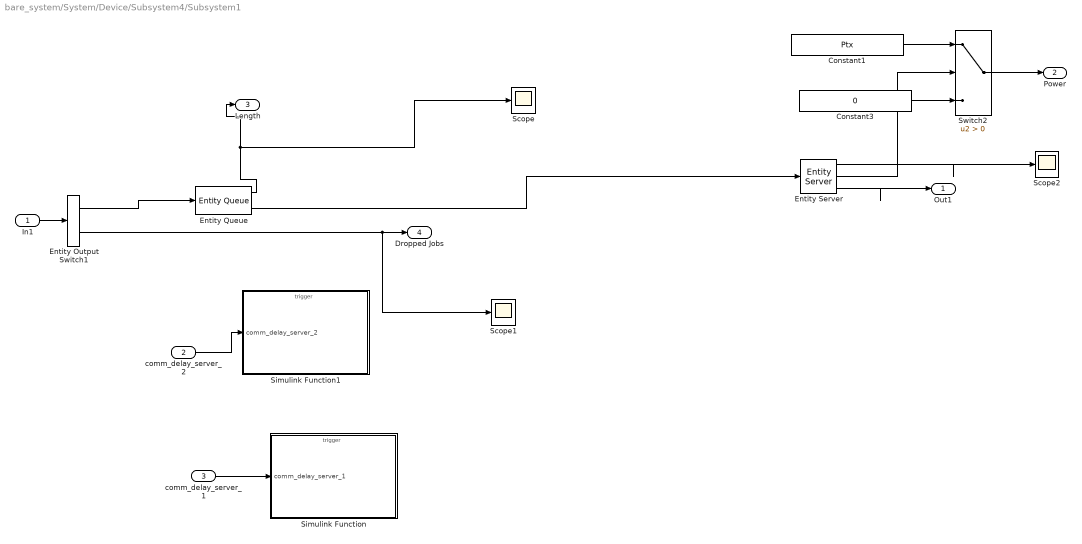
== system bare_system/System/Device/Subsystem4/Subsystem1 ==
  In1 : Inport
  comm_delay_server_2 : Inport  Port=2
  comm_delay_server_1 : Inport  Port=3
  Constant1 : Constant  Value=Ptx
  Constant3 : Constant  Value=0
  Entity Output Switch1 : EntityOutputSwitch  InputPortMessageModes=m  OutputPortMessageModes=m,m  SwitchAttributeName=platform
  Entity Queue : EntityQueue  InputPortMessageModes=m  OutputPortMessageModes=n,m  Capacity=20  NumberEntitiesInBlock=on
      settings: OutputPortMap=o1,o5
  Entity Server : EntityServer  InputPortMessageModes=m  OutputPortMessageModes=n,n,m  Capacity=1  ServiceTimeSource=MATLAB action  ServiceTimeAction=|  AverageWait=on  Utilization=on
      | % dt = rand(1,1);
      | 
      | wl=entity.size;
      | c_t=comm_time();
      | c_t2=comm_time2();
      | if(entity.platform==2)
      |     dt=wl/c_t;
      | else
      |     dt=wl/c_t2;
      | end
      settings: OutputPortMap=o4,o5,o9
  Scope : Scope
  Scope1 : Scope
  Scope2 : Scope
  Simulink Function : Subsystem  TreatAsAtomicUnit=on
  Simulink Function1 : Subsystem  TreatAsAtomicUnit=on
  Switch2 : Switch  Criteria=u2 > Threshold
  Out1 : Outport  VectorParamsAs1DForOutWhenUnconnected=on
  Power : Outport  Port=2  SampleTime=sample_time  VectorParamsAs1DForOutWhenUnconnected=on
  "Length " : Outport  Port=3  VectorParamsAs1DForOutWhenUnconnected=on
  Dropped Jobs : Outport  Port=4  VectorParamsAs1DForOutWhenUnconnected=on
  wires:
  Entity Server/3 -> Out1/1
  Switch2/1 -> Power/1
  Entity Server/2 -> Switch2/2
  Constant1/1 -> Switch2/1
  Constant3/1 -> Switch2/3
  Entity Queue/1 -> Scope/1, "Length "/1
  Entity Queue/2 -> Entity Server/1
  comm_delay_server_1/1 -> Simulink Function/1(comm_delay_server_1)
  comm_delay_server_2/1 -> Simulink Function1/1(comm_delay_server_2)
  Entity Output Switch1/2 -> Scope1/1, Dropped Jobs/1
  In1/1 -> Entity Output Switch1/1
  Entity Output Switch1/1 -> Entity Queue/1
  Entity Server/1 -> Scope2/1

== system bare_system/System/Reward Calculation /individual_rewards/Subsystem1 ==
  In2 : Inport
  Bus Selector2 : BusSelector  OutputSignals=encryptionLevel,integrityLevel,id
  Constant4 : Constant  Value=0
  Gain : Gain
  Subsystem : Subsystem
  Subsystem1 : Subsystem
  Subtract3 : Sum
  Switch5 : Switch  Criteria=u2 > Threshold
  alpha1 : Constant  Value=l1_cf
  alpha2 : Constant  Value=l1_ig
  Out1 : Outport  VectorParamsAs1DForOutWhenUnconnected=on
  wires:
  alpha2/1 -> Subsystem/1(Lambda)
  alpha1/1 -> Subsystem1/1(Lambda)
  Subsystem/1(P) -> Subtract3/2
  Constant4/1 -> Switch5/3
  Gain/1 -> Switch5/1  "Risk"
  Subtract3/1 -> Gain/1
  Bus Selector2/1 -> Subsystem1/2(SecurityLevel)  "<encryptionLevel>"
  Bus Selector2/2 -> Subsystem/2(SecurityLevel)  "<integrityLevel>"
  Bus Selector2/3 -> Switch5/2  "<id>"
  Subsystem1/1(P) -> Subtract3/1
  In2/1 -> Bus Selector2/1
  Switch5/1 -> Out1/1

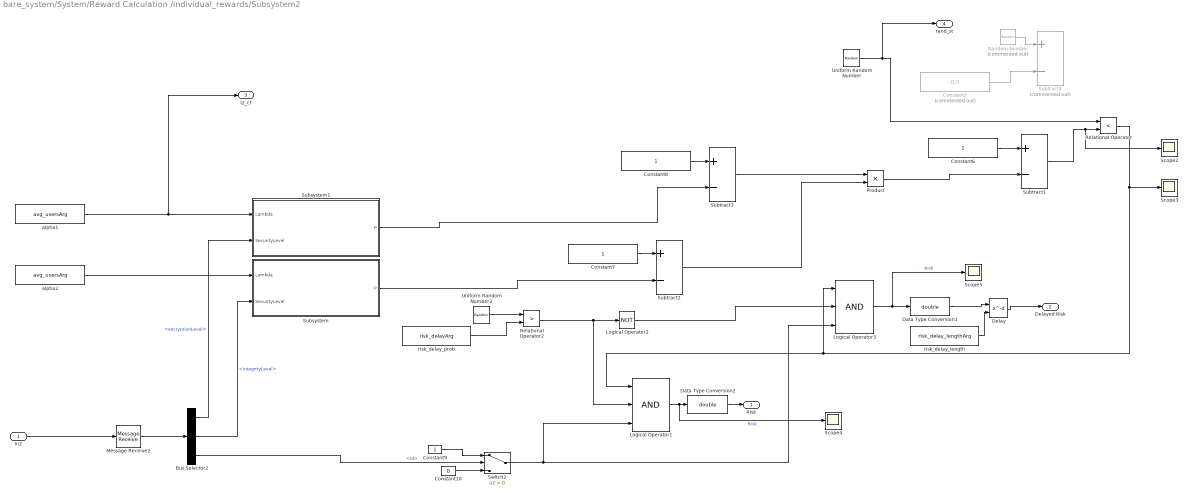
== system bare_system/System/Reward Calculation /individual_rewards/Subsystem2 ==
  In2 : Inport
  Bus Selector2 : BusSelector  OutputSignals=encryptionLevel,integrityLevel,id
  Constant10 : Constant  Value=0
  Constant2 : Constant  Commented=on  Value=0.5
  Constant{6..9} (4 alike) : Constant
  Data Type Conversion1 : DataTypeConversion  OutDataTypeStr=double
  Data Type Conversion2 : DataTypeConversion  OutDataTypeStr=double
  Delay : Delay  DelayLengthSource=Input port  DelayLength=interval  InitialCondition=0
      settings: InputPortMap=u0,p1
  Logical Operator1 : Logic  Inputs=3  AllPortsSameDT=off  OutDataTypeStr=boolean
  Logical Operator2 : Logic  Operator=NOT  AllPortsSameDT=off  OutDataTypeStr=boolean
  Logical Operator3 : Logic  Inputs=3  AllPortsSameDT=off  OutDataTypeStr=boolean
  Message Receive2 : MessageReceive  InputPortMessageModes=m  ValueSourceWhenQueueIsEmpty=Use initial value  SampleTime=0.1
      settings: OutputPortMap=o1
  Product : Product
  Random Number : RandomNumber  Commented=on  Variance=0.1  SampleTime=sample_time
  Relational Operator : RelationalOperator  Operator=<  OutDataTypeStr=boolean  RndMeth=Simplest
  Relational Operator2 : RelationalOperator  Operator=>  OutDataTypeStr=boolean  RndMeth=Simplest
  Scope{2..5} (4 alike) : Scope
  Subsystem : Subsystem
  Subsystem1 : Subsystem
  Subtract1 : Sum  Inputs=+-
  Subtract2 : Sum  Inputs=+-
  Subtract3 : Sum  Inputs=+-
  Subtract4 : Sum  Commented=on  Inputs=+-
  Switch2 : Switch  Criteria=u2 > Threshold
  Uniform Random Number : UniformRandomNumber  Minimum=0  SampleTime=interval
  Uniform Random Number2 : UniformRandomNumber  Minimum=0  Seed=1  SampleTime=0.1
  alpha1 : Constant  Value=avg_usersArg
  alpha2 : Constant  Value=avg_usersArg
  risk_delay_length : Constant  Value=risk_delay_lengthArg
  risk_delay_prob : Constant  Value=risk_delayArg
  Risk : Outport  VectorParamsAs1DForOutWhenUnconnected=on
  Delayed Risk : Outport  Port=2  VectorParamsAs1DForOutWhenUnconnected=on
  l2_cf : Outport  Port=3  VectorParamsAs1DForOutWhenUnconnected=on
  rand_st : Outport  Port=4  VectorParamsAs1DForOutWhenUnconnected=on
  wires:
  In2/1 -> Message Receive2/1
  Bus Selector2/3 -> Switch2/2  "<id>"
  Bus Selector2/2 -> Subsystem/2(SecurityLevel)  "<integrityLevel>"
  Bus Selector2/1 -> Subsystem1/2(SecurityLevel)  "<encryptionLevel>"
  alpha1/1 -> l2_cf/1, Subsystem1/1(Lambda)
  alpha2/1 -> Subsystem/1(Lambda)
  Subsystem/1(P) -> Subtract2/2
  Uniform Random Number2/1 -> Relational Operator2/1
  risk_delay_prob/1 -> Relational Operator2/2
  Relational Operator2/1 -> Logical Operator2/1, Logical Operator1/2
  Message Receive2/1 -> Bus Selector2/1
  Logical Operator1/1 -> Scope4/1, Data Type Conversion2/1  "Risk"
  Constant8/1 -> Subtract3/1
  Subsystem1/1(P) -> Subtract3/2
  Subtract3/1 -> Product/1
  Constant6/1 -> Subtract1/1
  Product/1 -> Subtract1/2
  Constant7/1 -> Subtract2/1
  Subtract2/1 -> Product/2
  Subtract1/1 -> Scope2/1, Relational Operator/2
  Relational Operator/1 -> Scope3/1, Logical Operator3/1, Logical Operator1/1
  Constant9/1 -> Switch2/1
  Constant10/1 -> Switch2/3
  Switch2/1 -> Logical Operator1/3, Logical Operator3/3
  Logical Operator2/1 -> Logical Operator3/2
  Logical Operator3/1 -> Scope5/1, Data Type Conversion1/1  "Risk"
  Delay/1 -> Delayed Risk/1
  Data Type Conversion1/1 -> Delay/1
  Random Number/1 -> Subtract4/1
  Constant2/1 -> Subtract4/2
  Uniform Random Number/1 -> rand_st/1, Relational Operator/1
  Data Type Conversion2/1 -> Risk/1
  risk_delay_length/1 -> Delay/2

== system bare_system/System/Device/Subsystem4/Subsystem1/Simulink Function ==
  comm_delay_server_1 : Inport
  comm_time : TriggerPort  TriggerType=function-call  IsSimulinkFunction=on  FunctionName=comm_time  FunctionVisibility=scoped  VariantControl=(inherit)
  MATLAB Function : MATLAB Function  TreatAsAtomicUnit=on
  encryptionLevel : ArgOut  DisableCoverage=on  ArgumentName=c_t
  wires:
  MATLAB Function/1(c_t) -> encryptionLevel/1
  comm_delay_server_1/1 -> MATLAB Function/1(u)

== system bare_system/System/Device/Subsystem4/Subsystem1/Simulink Function1 ==
  comm_delay_server_2 : Inport
  comm_time2 : TriggerPort  TriggerType=function-call  IsSimulinkFunction=on  FunctionName=comm_time2  FunctionVisibility=scoped  VariantControl=(inherit)
  MATLAB Function : MATLAB Function  TreatAsAtomicUnit=on
  c_t : ArgOut  DisableCoverage=on  ArgumentName=c_t
  wires:
  MATLAB Function/1(c_t) -> c_t/1
  comm_delay_server_2/1 -> MATLAB Function/1(u)

== system bare_system/System/Reward Calculation /individual_rewards/Subsystem1/Subsystem ==
  Lambda : Inport
  SecurityLevel : Inport  Port=2
  Constant8 : Constant
  Constant9 : Constant
  Divide3 : Product  Inputs=**
  Log2 : Math  SaturateOnIntegerOverflow=on
  Subtract3 : Sum  Inputs=+-
  Subtract4 : Sum  Inputs=+-
  Unary Minus : UnaryMinus
  P : Outport  VectorParamsAs1DForOutWhenUnconnected=on
  wires:
  SecurityLevel/1 -> Subtract3/2
  Divide3/1 -> Unary Minus/1  "SINR"
  Subtract3/1 -> Divide3/1
  Constant9/1 -> Subtract4/1
  Constant8/1 -> Subtract3/1
  Log2/1 -> Subtract4/2
  Subtract4/1 -> P/1
  Unary Minus/1 -> Log2/1
  Lambda/1 -> Divide3/2

== system bare_system/System/Reward Calculation /individual_rewards/Subsystem1/Subsystem1 ==
  Lambda : Inport
  SecurityLevel : Inport  Port=2
  Constant8 : Constant
  Constant9 : Constant
  Divide3 : Product  Inputs=**
  Log2 : Math  SaturateOnIntegerOverflow=on
  Subtract3 : Sum  Inputs=+-
  Subtract4 : Sum  Inputs=+-
  Unary Minus : UnaryMinus
  P : Outport  VectorParamsAs1DForOutWhenUnconnected=on
  wires:
  Lambda/1 -> Divide3/2
  Unary Minus/1 -> Log2/1
  Subtract4/1 -> P/1
  Log2/1 -> Subtract4/2
  Constant8/1 -> Subtract3/1
  Constant9/1 -> Subtract4/1
  Subtract3/1 -> Divide3/1
  Divide3/1 -> Unary Minus/1  "SINR"
  SecurityLevel/1 -> Subtract3/2

== system bare_system/System/Reward Calculation /individual_rewards/Subsystem2/Subsystem ==
  Lambda : Inport
  SecurityLevel : Inport  Port=2
  Constant8 : Constant
  Constant9 : Constant
  Divide3 : Product  Inputs=**
  Log2 : Math  SaturateOnIntegerOverflow=on
  Subtract3 : Sum  Inputs=+-
  Subtract4 : Sum  Inputs=+-
  Unary Minus : UnaryMinus
  P : Outport  VectorParamsAs1DForOutWhenUnconnected=on
  wires:
  Lambda/1 -> Divide3/2
  Unary Minus/1 -> Log2/1
  Subtract4/1 -> P/1
  Log2/1 -> Subtract4/2
  Constant8/1 -> Subtract3/1
  Constant9/1 -> Subtract4/1
  Subtract3/1 -> Divide3/1
  Divide3/1 -> Unary Minus/1  "SINR"
  SecurityLevel/1 -> Subtract3/2

== system bare_system/System/Reward Calculation /individual_rewards/Subsystem2/Subsystem1 ==
  Lambda : Inport
  SecurityLevel : Inport  Port=2
  Constant8 : Constant
  Constant9 : Constant
  Divide3 : Product  Inputs=**
  Log2 : Math  SaturateOnIntegerOverflow=on
  Subtract3 : Sum  Inputs=+-
  Subtract4 : Sum  Inputs=+-
  Unary Minus : UnaryMinus
  P : Outport  VectorParamsAs1DForOutWhenUnconnected=on
  wires:
  SecurityLevel/1 -> Subtract3/2
  Divide3/1 -> Unary Minus/1  "SINR"
  Subtract3/1 -> Divide3/1
  Constant9/1 -> Subtract4/1
  Constant8/1 -> Subtract3/1
  Log2/1 -> Subtract4/2
  Subtract4/1 -> P/1
  Unary Minus/1 -> Log2/1
  Lambda/1 -> Divide3/2

== matlab function System/Device/Simulink Function3/MATLAB Function ==
  data: l1 input double; dt output double; total_time input double; interval input double; j1_in output double; curr_time input double; seed input double
function [dt,j1_in] = fcn(l1,total_time,interval,curr_time,seed)

% This function generates the events for the episode. l1, l2 are the rate
% of job arrivals for two types of jobs j1 and j2. dt1,dt2 are the
% interarrival times. j1_in, j2_in are the total jobs in the current
% interval.

persistent dts1;
persistent idx1;
persistent e_ins1;


if(isempty(dts1))
%     only called at the beginning 
    rng(seed);  
    [~,dts1,e_ins1]=createEvents(l1,total_time+1,interval);
    idx1=0;
    
end
% when l1 is close to 0 or 0, there can be no event in the whole simulation
% in such case dts1 is empty. This should protect against it and allow safe
% running.
if(isempty(dts1))
    
    dt=total_time+1;
    j1_in=0;
else
idx1=min(idx1+1,numel(dts1));

dt=dts1(idx1);
idx_1=floor(curr_time/interval)+1;
j1_in=e_ins1(idx_1);
end

== matlab function System/Device/Simulink Function1/MATLAB Function ==
  data: idx output double
function idx = fcn()

persistent id;

if isempty(id)
    id=0;
end

id=id+1;
idx=(id);

== matlab function System/Device/Simulink Function7/MATLAB Function2 ==
  data: encryptionLevel input double; encryptionLevel output double; integrityLevel input double; encryptionWorkloadPerBit output double; integrityLevel output double; integrityWorkloadPerBit output double
function [encryptionLevel, encryptionWorkloadPerBit, integrityLevel, integrityWorkloadPerBit] = selectSecurity(encryptionLevel,integrityLevel)
%options =2
%action =0.2

Mbtob=1024*1024;

if(encryptionLevel<=0)
    rate=inf;
    encryptionLevel=0;
elseif(encryptionLevel<=0.32)
    rate=37.17;
elseif(encryptionLevel<=0.53)
    rate=33.03;
elseif(encryptionLevel<=0.56)
    rate=20.87;
elseif(encryptionLevel<=0.85)
    rate=13.83;
elseif(encryptionLevel<=1)
    rate=11.76;
else
    rate=inf;
end
% switch(encryptionLevel)
%     case 1
%         rate=11.76;
%         
%     case 0.85
%         rate=13.83;
%         
%     case 0.56
%         rate=20.87;
%         
%     case 0.53 
%         rate=33.03;
%         
%     case 0.32
%         rate=37.17;
%         
%     otherwise
%         rate=inf;
%         encryptionLevel=0;
%         
% end
encryptionWorkloadPerBit=1/(rate*Mbtob);
if(integrityLevel<=0)
    rate=inf;
    integrityLevel=0;
elseif(integrityLevel<=0.44)
    rate=172.41;
elseif(integrityLevel<=0.63)
    rate=119.05;
elseif(integrityLevel<=0.69)
    rate=109.89;
elseif(integrityLevel<=0.75)
    rate=101.01;
elseif(integrityLevel<=1)
    rate=75.76;
else
    rate=inf;
end
% switch(integrityLevel)
%     case 1
%         rate=75.75;
%         
%     case 0.75
%         rate=101.01;
%     case 0.69
%         rate=109.89;
% 
%     case 0.63
%         rate=119.05;
%         
%     case 0.44
%         rate=172.41;
%         
%     otherwise
%         rate=inf;
%         integrityLevel=0;
%         
% end
integrityWorkloadPerBit=1/(rate*Mbtob);
    

% assert(selection<=options);

== matlab function System/Device/Simulink Function4/MATLAB Function ==
  data: l2 input double; total_time input double; interval input double; dt output double; j2_in output double; curr_time input double
function [dt,j2_in] = fcn(l2,total_time,interval,curr_time)

% This function generates the events for the episode. l1, l2 are the rate
% of job arrivals for two types of jobs j1 and j2. dt1,dt2 are the
% interarrival times. j1_in, j2_in are the total jobs in the current
% interval.



persistent dts2;
persistent idx2;
persistent e_ins2;


if(isempty(dts2))
    
    [~,dts2,e_ins2]=createEvents(l2,total_time+1,interval);
    idx2=0;
    
end
% when l2 is close to 0 or 0, there can be no event in the whole simulation
% in such case dts1 is empty. This should protect against it and allow safe
% running.
if(isempty(dts2))
    
    dt=total_time+1;
    j2_in=0;
else

idx2=min(idx2+1,numel(dts2));

dt=dts2(idx2);
idx_2=floor(curr_time/interval)+1;
j2_in=e_ins2(idx_2);



end

== matlab function System/Device/Simulink Function8/MATLAB Function2 ==
  data: action1 input double; platform output double; action2 input double
function platform = offloadSelection(action1,action2)
%options =2
%action =0.2
r=rand()*2; %range 0-2



if(r<=action1)
    platform=1;
elseif(r<=action1+action2)
    
    platform=2;
else
    platform=3;
end

% assert(selection<=options);

== matlab function System/Device/Simulink Function5/MATLAB Function2 ==
  data: action1 input double; platform output double
function platform = job1decision(action1)
%options =2
%action =0.2
r=rand(); %range 0-2
% 
% % action1=action1;
% % action2=action2*2;
% 
if(r<=action1)
    platform=1;
% elseif(r<=action1+action2)
%     
%     platform=2;
else
    platform=2;
end
% platform=action1;
% assert(selection<=options);

== matlab function System/MATLAB Function1 ==
  data: no_users output double; randomSeenArg input double; lower_limit input double; upper_limit input double
function no_users = fcn(randomSeenArg,lower_limit,upper_limit)
%options =2
%action =0.2
% if(nt_type==1) %best
%     no_users=round(normrnd(5,2.5));
% elseif(nt_type==2) %medium
%     no_users=round(normrnd(25,2.5));
% else
%     no_users=round(normrnd(70,2.5));
% end
persistent rngInit;

if isempty(rngInit)
    rng(randomSeenArg);
    rngInit=true;
end

no_users = (upper_limit-lower_limit).*rand(1,1) + lower_limit;

no_users=min(max(1,no_users),100);

% assert(selection<=options);

== matlab function System/Device/Subsystem4/Subsystem1/Simulink Function/MATLAB Function ==
  data: u input double; c_t output double
function c_t = comm_time(u)


c_t=u;

== matlab function System/Device/Subsystem4/Subsystem1/Simulink Function1/MATLAB Function ==
  data: u input double; c_t output double
function c_t = comm_time2(u)


c_t=u;

== matlab function System/Reward Calculation /Integrator/MATLAB Function ==
  data: event input double; count output double; reset input double; prev_count output double
function [count,prev_count] = fcn(event,reset)
persistent previous_count previous_reset


if(isempty(previous_reset))
    previous_reset=0;
end
if(isempty(previous_count))
    previous_count=0;
end
count=event-previous_count;
prev_count=previous_count;
if(reset==0&&previous_reset==1)
    previous_count=event;
end



previous_reset=reset;
